simulink model "sxema"  (R2013a)
settings: Solver=ode3  StartTime=0.0  StopTime=0.6  FixedStep=0.001  RelTol=1e-3
settings Model: Creator=Huy Hung  LastModifiedBy=Sion

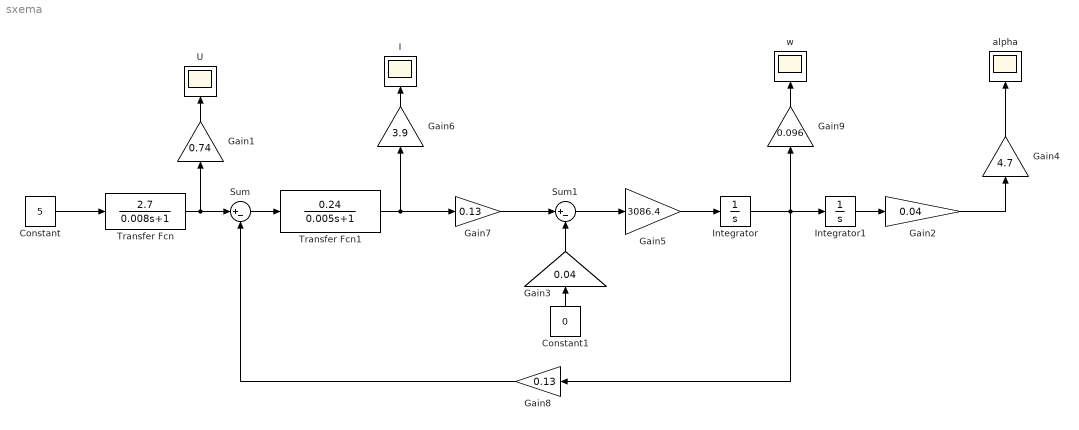
== system sxema ==
  Constant : Constant  Value=5
  Constant1 : Constant  Value=0
  Gain1 : Gain  Gain=0.74
  Gain2 : Gain  Gain=0.04
  Gain3 : Gain  Gain=0.04
  Gain4 : Gain  Gain=4.7
  Gain5 : Gain  Gain=3086.4
  Gain6 : Gain  Gain=3.9
  Gain7 : Gain  Gain=0.13
  Gain8 : Gain  Gain=0.13
  Gain9 : Gain  Gain=0.096
  I : Scope
      settings: SaveName=I
  Integrator : Integrator
  Integrator1 : Integrator
  Sum : Sum  Inputs=|+-
  Sum1 : Sum  Inputs=|+-
  Transfer Fcn : TransferFcn  Numerator=[2.7]  Denominator=[0.008 1]
  Transfer Fcn1 : TransferFcn  Numerator=[0.24]  Denominator=[0.005 1]
  U : Scope
      settings: SaveName=U
  alpha : Scope
      settings: SaveName=alpha
  w : Scope
      settings: SaveName=w
  wires:
  Constant/1 -> Transfer Fcn/1
  Transfer Fcn/1 -> Sum/1, Gain1/1
  Sum/1 -> Transfer Fcn1/1
  Gain5/1 -> Integrator/1
  Integrator1/1 -> Gain2/1
  Gain2/1 -> Gain4/1
  Gain4/1 -> alpha/1
  Gain7/1 -> Sum1/1
  Sum1/1 -> Gain5/1
  Gain3/1 -> Sum1/2
  Constant1/1 -> Gain3/1
  Gain8/1 -> Sum/2
  Gain1/1 -> U/1
  Transfer Fcn1/1 -> Gain6/1, Gain7/1
  Gain6/1 -> I/1
  Integrator/1 -> Gain9/1, Gain8/1, Integrator1/1
  Gain9/1 -> w/1
